simulink model "ctrl"  (R2018a)
settings: Solver=FixedStepDiscrete  StartTime=0.0  StopTime=0.1  RelTol=1e-3  EnableMultiTasking=on
undefined symbols (not defined in the file): AutoCalSt, Cfg_AutoCalEnbl, Cfg_EnblLoadObs, Cfg_IfbkCtrlBW, Cfg_SpdCtrlBW, Cfg_SpdSnsSrc, DiscIntNeverNeededParam, DistObs_K1, DistObs_K2, DistObs_K3, EncResDeg, MotorParams, MtrCtrlMd, SmDiff_Ki, SmDiff_Kp, TsFast
libraries: ctrl_lib x9, simulink_extras x4, simulink x3, adrc_lib x1
settings Model: PauseTimes=0.1  Creator=uids8840  LastModifiedBy=elrobotista
settings SolverCC: AutoInsertRateTranBlk=on
settings DataIOCC: SaveOutput=off  SignalLogging=off  DSMLogging=off  SaveTime=off
settings OptimizationCC: UseFloatMulNetSlope=on  PassReuseOutputArgsAs=Individual arguments  ZeroExternalMemoryAtStartup=off  ZeroInternalMemoryAtStartup=off  NoFixptDivByZeroProtection=on  EfficientFloat2IntCast=on  LifeSpan=1
settings DebuggingCC: ParameterTunabilityLossMsg=error
settings HardwareCC: ProdBitPerPointer=32  ProdBitPerSizeT=32  ProdBitPerPtrDiffT=32  ProdLargestAtomicInteger=Long  ProdLargestAtomicFloat=Double  ProdWordSize=32  ProdHWDeviceType=ARM Compatible->ARM Cortex
settings ModelReferenceCC: ModelReferenceNumInstancesAllowed=Single
settings SFSimCC: MATLABDynamicMemAlloc=off
settings RTWCC: SystemTargetFile=ert.tlc  GenCodeOnly=on  PackageGeneratedCodeAndArtifacts=on  PackageName=mtrctl  TemplateMakefile=ert_default_tmf  GenerateReport=on  IncludeHyperlinkInReport=on  LaunchReport=on  GenerateTraceInfo=on  GenerateTraceReport=on  GenerateTraceReportSl=on  GenerateTraceReportSf=on  GenerateTraceReportEml=on  GenerateCodeMetricsReport=on
settings CodeAppCC: ForceParamTrailComments=on  IgnoreCustomStorageClasses=off  OperatorAnnotations=on  SimulinkDataObjDesc=on  SFDataObjDesc=on  CustomSymbolStrGlobalVar=rt$N$M  CustomSymbolStrType=$N$M  CustomSymbolStrFcn=$N$M$F  CustomSymbolStrMacro=$N$M  InsertBlockDesc=on
settings ERTTargetCC: TargetLangStandard=C99 (ISO)  GenerateFullHeader=off  IncludeMdlTerminateFcn=off  CombineSignalStateStructs=on  SuppressErrorStatus=on  ERTCustomFileBanners=off  SupportAbsoluteTime=off  SupportNonFinite=off  SupportComplex=off  ERTCustomFileTemplate=example_file_process.tlc

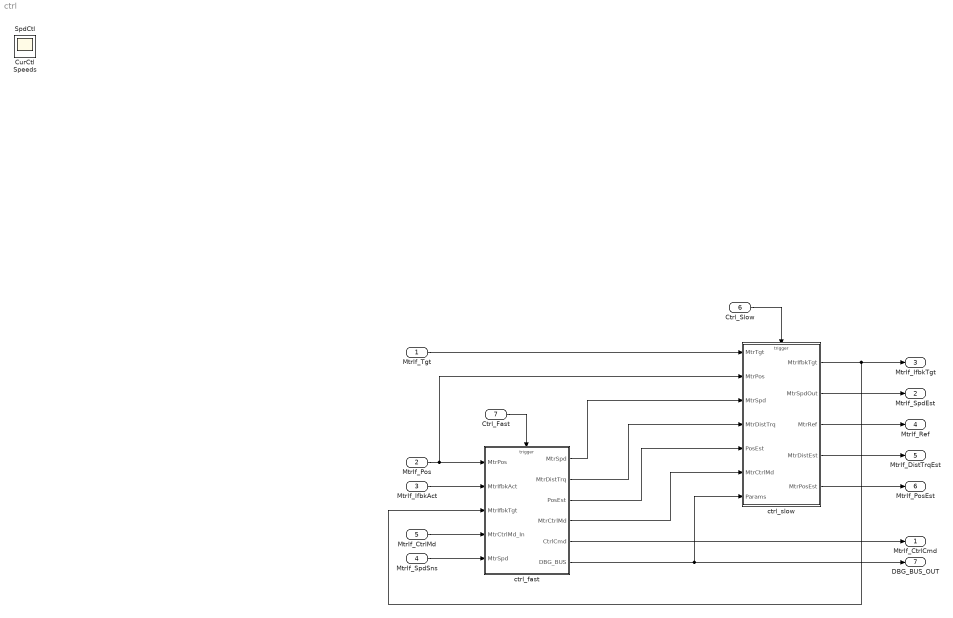
== system ctrl ==
  MtrIf_Tgt : Inport  OutDataTypeStr=single
  MtrIf_Pos : Inport  Port=2  OutDataTypeStr=single
  MtrIf_IfbkAct : Inport  Port=3  OutDataTypeStr=single
  MtrIf_SpdSns : Inport  Port=4
  MtrIf_CtrlMd : Inport  Port=5  OutDataTypeStr=Enum: MtrCtrlMd
  Ctrl_Slow : Inport  Port=6  OutputFunctionCall=on
  Ctrl_Fast : Inport  Port=7  OutputFunctionCall=on
  ctrl_fast : Subsystem  TreatAsAtomicUnit=on  SystemSampleTime=1/30e3
      settings: RTWFcnNameOpts=Use subsystem name  RTWFileNameOpts=Use subsystem name  FunctionInterfaceSpec=Allow arguments
  ctrl_slow : Subsystem  TreatAsAtomicUnit=on  SystemSampleTime=1/1e3
      settings: RTWFcnNameOpts=Use subsystem name  RTWFileNameOpts=Use function name  FunctionInterfaceSpec=Allow arguments
  MtrIf_CtrlCmd : Outport
  MtrIf_SpdEst : Outport  Port=2
  MtrIf_IfbkTgt : Outport  Port=3
  MtrIf_Ref : Outport  Port=4
  MtrIf_DistTrqEst : Outport  Port=5
  MtrIf_PosEst : Outport  Port=6
  DBG_BUS_OUT : Outport  Port=7  OutDataTypeStr=Bus: DBG_BUS  BusOutputAsStruct=on
  CurCtl : Scope
  SpdCtl : Scope
  Speeds : Scope
  wires:
  ctrl_fast/1(MtrSpd) -> ctrl_slow/3(MtrSpd)
  Ctrl_Slow/1 -> ctrl_slow/Trigger
  Ctrl_Fast/1 -> ctrl_fast/Trigger
  MtrIf_IfbkAct/1 -> ctrl_fast/2(MtrIfbkAct)
  MtrIf_Pos/1 -> ctrl_fast/1(" MtrPos"), ctrl_slow/2(MtrPos)
  ctrl_slow/2(MtrSpdOut) -> MtrIf_SpdEst/1
  ctrl_slow/1(MtrIfbkTgt) -> MtrIf_IfbkTgt/1, ctrl_fast/3(MtrIfbkTgt)
  MtrIf_Tgt/1 -> ctrl_slow/1(MtrTgt)
  ctrl_slow/3(MtrRef) -> MtrIf_Ref/1
  ctrl_slow/4(MtrDistEst) -> MtrIf_DistTrqEst/1
  ctrl_slow/5(MtrPosEst) -> MtrIf_PosEst/1
  ctrl_fast/5(CtrlCmd) -> MtrIf_CtrlCmd/1
  ctrl_fast/2(MtrDistTrq) -> ctrl_slow/4(MtrDistTrq)
  ctrl_fast/3(PosEst) -> ctrl_slow/5(PosEst)
  MtrIf_CtrlMd/1 -> ctrl_fast/4(MtrCtrlMd_In)
  MtrIf_SpdSns/1 -> ctrl_fast/5(" MtrSpd")
  ctrl_fast/4(MtrCtrlMd) -> ctrl_slow/6(MtrCtrlMd)
  ctrl_fast/6(DBG_BUS) -> ctrl_slow/7(Params), DBG_BUS_OUT/1

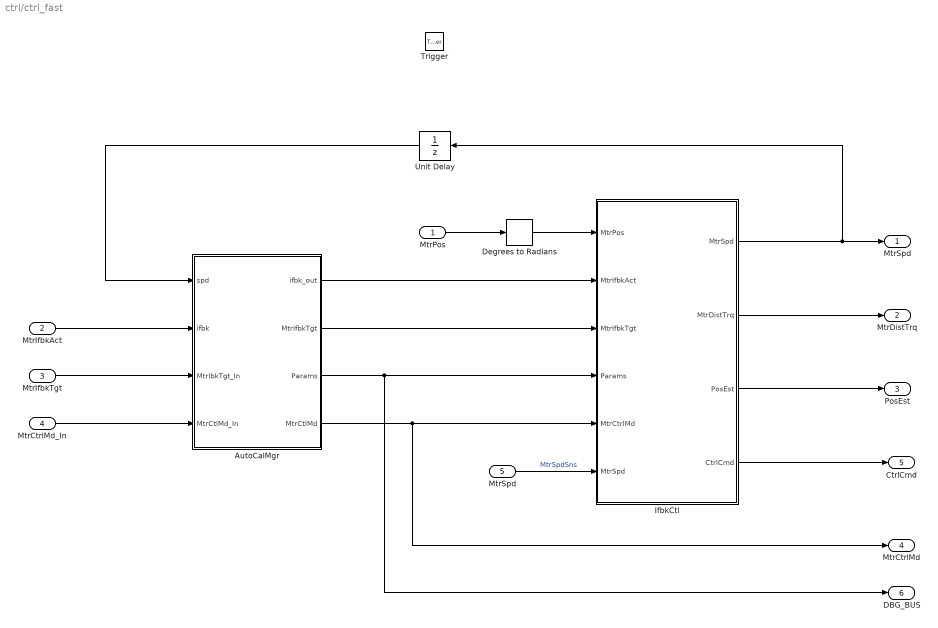
== system ctrl/ctrl_fast ==
  " MtrPos" : Inport
  MtrIfbkAct : Inport  Port=2
  MtrIfbkTgt : Inport  Port=3
  MtrCtrlMd_In : Inport  Port=4
  " MtrSpd" : Inport  Port=5
  Trigger : TriggerPort  TriggerType=function-call  VariantControl=Variant  PortDimensions=1
  AutoCalMgr : Subsystem
  Degrees to Radians : simulink_extras/Transformations/Degrees to Radians
  IfbkCtl : Subsystem
  Unit Delay : UnitDelay  SampleTime=-1
  MtrSpd : Outport
  MtrDistTrq : Outport  Port=2
  PosEst : Outport  Port=3
  MtrCtrlMd : Outport  Port=4
  CtrlCmd : Outport  Port=5
  DBG_BUS : Outport  Port=6  OutDataTypeStr=Bus: DBG_BUS
  wires:
  " MtrSpd"/1 -> IfbkCtl/6(" MtrSpd")  "MtrSpdSns"
  IfbkCtl/2(MtrDistTrq) -> MtrDistTrq/1
  IfbkCtl/4(CtrlCmd) -> CtrlCmd/1
  MtrIfbkAct/1 -> AutoCalMgr/2(ifbk)
  MtrIfbkTgt/1 -> AutoCalMgr/3(MtrIbkTgt_In)
  AutoCalMgr/1(ifbk_out) -> IfbkCtl/2(MtrIfbkAct)
  AutoCalMgr/2(MtrIfbkTgt) -> IfbkCtl/3(MtrIfbkTgt)
  AutoCalMgr/4(MtrCtlMd) -> MtrCtrlMd/1, IfbkCtl/5(MtrCtrlMd)
  MtrCtrlMd_In/1 -> AutoCalMgr/4(MtrCtlMd_In)
  AutoCalMgr/3(Params) -> DBG_BUS/1, IfbkCtl/4(Params)
  IfbkCtl/1(MtrSpd) -> Unit Delay/1, MtrSpd/1
  Unit Delay/1 -> AutoCalMgr/1(spd)
  " MtrPos"/1 -> Degrees to Radians/1
  Degrees to Radians/1 -> IfbkCtl/1(" MtrPos")
  IfbkCtl/3(PosEst) -> PosEst/1

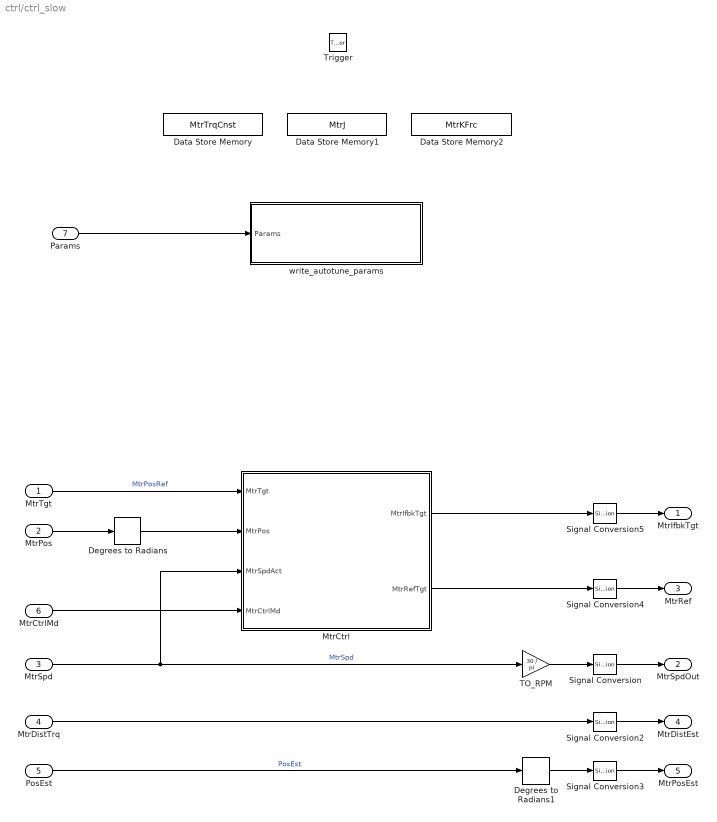
== system ctrl/ctrl_slow ==
  MtrTgt : Inport
  MtrPos : Inport  Port=2
  MtrSpd : Inport  Port=3
  MtrDistTrq : Inport  Port=4
  PosEst : Inport  Port=5
  MtrCtrlMd : Inport  Port=6
  Params : Inport  Port=7  OutDataTypeStr=Bus: DBG_BUS
  Trigger : TriggerPort  TriggerType=function-call  VariantControl=Variant  PortDimensions=1
  Data Store Memory : DataStoreMemory  DataStoreName=MtrTrqCnst  ReadBeforeWriteMsg=warning  WriteAfterWriteMsg=warning  WriteAfterReadMsg=warning  ShowAdditionalParam=off
  Data Store Memory1 : DataStoreMemory  DataStoreName=MtrJ  ReadBeforeWriteMsg=warning  WriteAfterWriteMsg=warning  WriteAfterReadMsg=warning  ShowAdditionalParam=off
  Data Store Memory2 : DataStoreMemory  DataStoreName=MtrKFrc  ReadBeforeWriteMsg=warning  WriteAfterWriteMsg=warning  WriteAfterReadMsg=warning  ShowAdditionalParam=off
  Degrees to Radians : simulink_extras/Transformations/Degrees to Radians
  Degrees to Radians1 : simulink_extras/Transformations/Degrees to Radians
  MtrCtrl : Subsystem
  Signal Conversion{,2..5} (5 alike) : SignalConversion  OverrideOpt=off
  TO_RPM : Gain  Gain=30 / pi
  write_autotune_params : Subsystem
  MtrIfbkTgt : Outport
  MtrSpdOut : Outport  Port=2
  MtrRef : Outport  Port=3
  MtrDistEst : Outport  Port=4
  MtrPosEst : Outport  Port=5
  wires:
  MtrCtrl/1(MtrIfbkTgt) -> Signal Conversion5/1
  Signal Conversion5/1 -> MtrIfbkTgt/1
  Signal Conversion/1 -> MtrSpdOut/1
  PosEst/1 -> Degrees to Radians1/1  "PosEst"
  Signal Conversion2/1 -> MtrDistEst/1
  Signal Conversion3/1 -> MtrPosEst/1
  Signal Conversion4/1 -> MtrRef/1
  MtrTgt/1 -> MtrCtrl/1(MtrTgt)  "MtrPosRef"
  MtrCtrlMd/1 -> MtrCtrl/4(MtrCtrlMd)
  MtrDistTrq/1 -> Signal Conversion2/1
  MtrPos/1 -> Degrees to Radians/1
  MtrCtrl/2(MtrRefTgt) -> Signal Conversion4/1
  Params/1 -> write_autotune_params/1(Params)
  Degrees to Radians/1 -> MtrCtrl/2(MtrPos)
  Degrees to Radians1/1 -> Signal Conversion3/1
  TO_RPM/1 -> Signal Conversion/1
  MtrSpd/1 -> MtrCtrl/3(MtrSpdAct), TO_RPM/1  "MtrSpd"

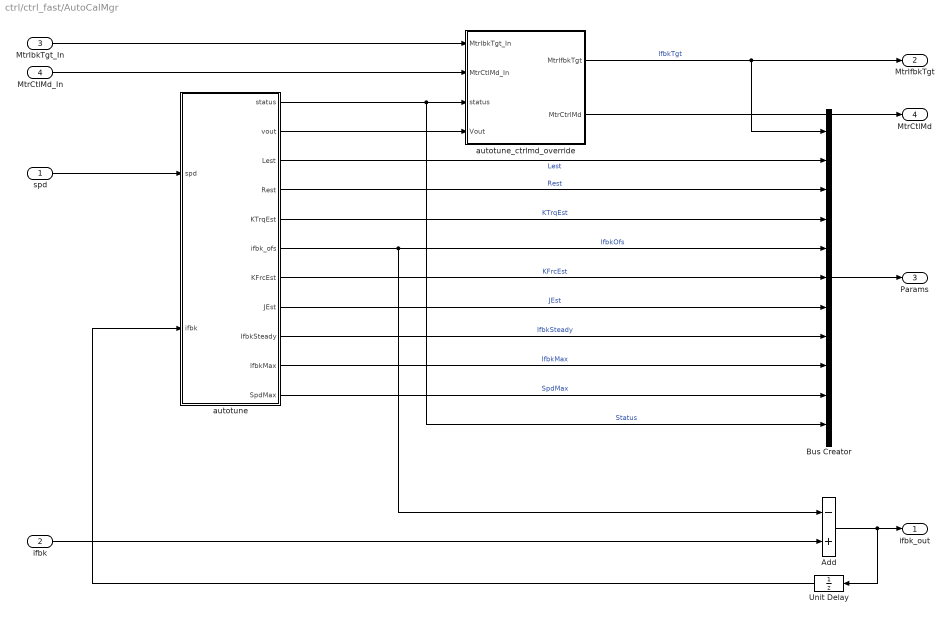
== system ctrl/ctrl_fast/AutoCalMgr ==
  spd : Inport
  ifbk : Inport  Port=2
  MtrIbkTgt_In : Inport  Port=3
  MtrCtlMd_In : Inport  Port=4
  Add : Sum  Inputs=-+
  Bus Creator : BusCreator  Inputs=11  OutDataTypeStr=Bus: DBG_BUS  NonVirtualBus=on
  Unit Delay : UnitDelay  SampleTime=-1
  autotune : Stateflow chart  TreatAsAtomicUnit=on
  autotune_ctrlmd_override : Subsystem
  ifbk_out : Outport
  MtrIfbkTgt : Outport  Port=2
  Params : Outport  Port=3
  MtrCtlMd : Outport  Port=4
  wires:
  MtrIbkTgt_In/1 -> autotune_ctrlmd_override/1(MtrIbkTgt_In)
  MtrCtlMd_In/1 -> autotune_ctrlmd_override/2(MtrCtlMd_In)
  autotune_ctrlmd_override/1(MtrIfbkTgt) -> Bus Creator/1, MtrIfbkTgt/1  "IfbkTgt"
  autotune_ctrlmd_override/2(MtrCtrlMd) -> MtrCtlMd/1
  autotune/1(status) -> Bus Creator/11, autotune_ctrlmd_override/3(status)  "Status"
  autotune/2(vout) -> autotune_ctrlmd_override/4(Vout)
  Bus Creator/1 -> Params/1
  ifbk/1 -> Add/2
  spd/1 -> autotune/1(spd)
  autotune/6(ifbk_ofs) -> Bus Creator/5, Add/1  "IfbkOfs"
  Add/1 -> Unit Delay/1, ifbk_out/1
  Unit Delay/1 -> autotune/2(ifbk)
  autotune/3(Lest) -> Bus Creator/2  "Lest"
  autotune/4(Rest) -> Bus Creator/3  "Rest"
  autotune/5(KTrqEst) -> Bus Creator/4  "KTrqEst"
  autotune/7(KFrcEst) -> Bus Creator/6  "KFrcEst"
  autotune/8(JEst) -> Bus Creator/7  "JEst"
  autotune/9(IfbkSteady) -> Bus Creator/8  "IfbkSteady"
  autotune/10(IfbkMax) -> Bus Creator/9  "IfbkMax"
  autotune/11(SpdMax) -> Bus Creator/10  "SpdMax"

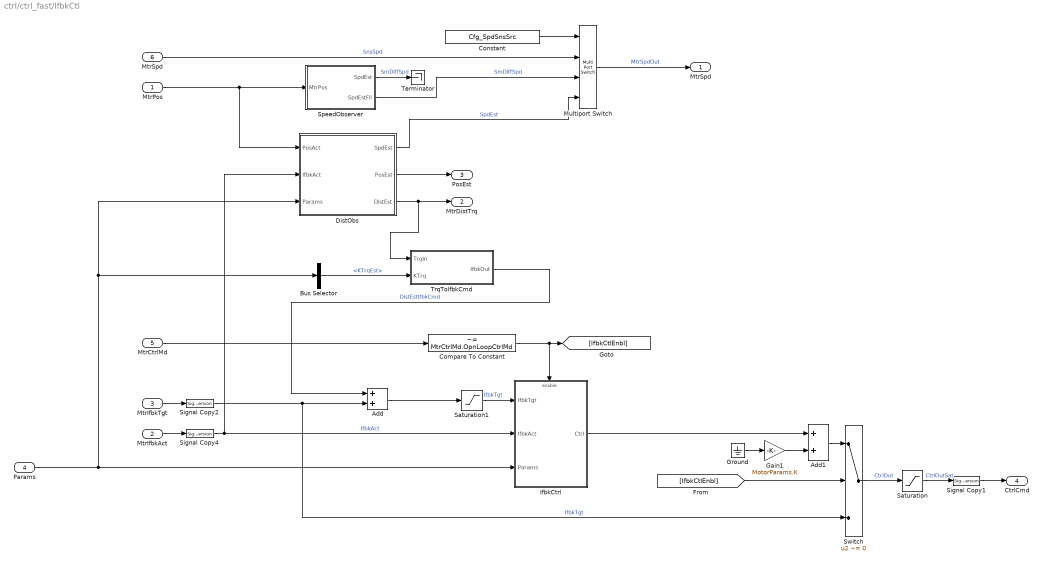
== system ctrl/ctrl_fast/IfbkCtl ==
  " MtrPos" : Inport
  MtrIfbkAct : Inport  Port=2
  MtrIfbkTgt : Inport  Port=3
  Params : Inport  Port=4
  MtrCtrlMd : Inport  Port=5
  " MtrSpd" : Inport  Port=6
  Add : Sum
  Add1 : Sum
  Bus Selector : BusSelector  OutputSignals=KTrqEst
  Compare To Constant : simulink/Logic and Bit Operations/Compare To Constant  relop=~=  const=MtrCtrlMd.OpnLoopCtrlMd  OutDataTypeStr=boolean
  Constant : Constant  Value=Cfg_SpdSnsSrc
  DistObs : Subsystem
  Gain1 : Gain  Gain=MotorParams.K
      settings: AttributesFormatString=%<Gain>
  Ground : Ground
  IfbkCtrl : Subsystem
  Multiport Switch : MultiPortSwitch  DataPortOrder=Zero-based contiguous  DiagnosticForDefault=None  zeroidx=on
  Saturation : Saturate  UpperLimit=12  LowerLimit=-12
  Saturation1 : Saturate  UpperLimit=0.6  LowerLimit=-0.6
  Signal Copy1 : SignalConversion  OverrideOpt=off
  Signal Copy2 : SignalConversion  OverrideOpt=off
  Signal Copy4 : SignalConversion  OverrideOpt=off
  SpeedObserver : Subsystem  RTWFcnName=SpdEst  RTWFileName=spdest
      settings: RTWFcnNameOpts=Use subsystem name  RTWFileNameOpts=Use subsystem name
  Switch : Switch  Criteria=u2 ~= 0
  Terminator : Terminator
  TrqToIfbkCmd : Subsystem
  MtrSpd : Outport
  MtrDistTrq : Outport  Port=2
  PosEst : Outport  Port=3
  CtrlCmd : Outport  Port=4
  wires:
  IfbkCtrl/1(Ctrl) -> Add1/1
  Compare To Constant/1 -> [IfbkCtlEnbl], IfbkCtrl/Enable
  MtrIfbkTgt/1 -> Signal Copy2/1
  MtrCtrlMd/1 -> Compare To Constant/1
  Add1/1 -> Switch/1
  Signal Copy4/1 -> DistObs/2(IfbkAct), IfbkCtrl/2(IfbkAct)  "IfbkAct"
  Gain1/1 -> Add1/2
  Multiport Switch/1 -> MtrSpd/1  "MtrSpdOut"
  Switch/1 -> Saturation/1  "CtrlOut"
  MtrIfbkAct/1 -> Signal Copy4/1
  " MtrSpd"/1 -> Multiport Switch/2  "SnsSpd"
  Constant/1 -> Multiport Switch/1
  [IfbkCtlEnbl] -> Switch/2
  Signal Copy2/1 -> Add/2, Switch/3  "IfbkTgt"
  SpeedObserver/2(SpdEstFil) -> Multiport Switch/3  "SmDiffSpd"
  " MtrPos"/1 -> DistObs/1(PosAct), SpeedObserver/1(MtrPos)
  Ground/1 -> Gain1/1
  Saturation/1 -> Signal Copy1/1  "CtrlOutSat"
  Signal Copy1/1 -> CtrlCmd/1
  Params/1 -> DistObs/3(Params), Bus Selector/1, IfbkCtrl/3(Params)
  SpeedObserver/1(SpdEst) -> Terminator/1  "SmDiffSpd"
  Saturation1/1 -> IfbkCtrl/1(IfbkTgt)  "IfbkTgt"
  TrqToIfbkCmd/1(IfbkOut) -> Add/1  "DistEstIfbkCmd"
  Add/1 -> Saturation1/1
  DistObs/3(DistEst) -> MtrDistTrq/1, TrqToIfbkCmd/1(TrqIn)
  DistObs/1(SpdEst) -> Multiport Switch/4  "SpdEst"
  DistObs/2(PosEst) -> PosEst/1
  Bus Selector/1 -> TrqToIfbkCmd/2(KTrq)  "<KTrqEst>"

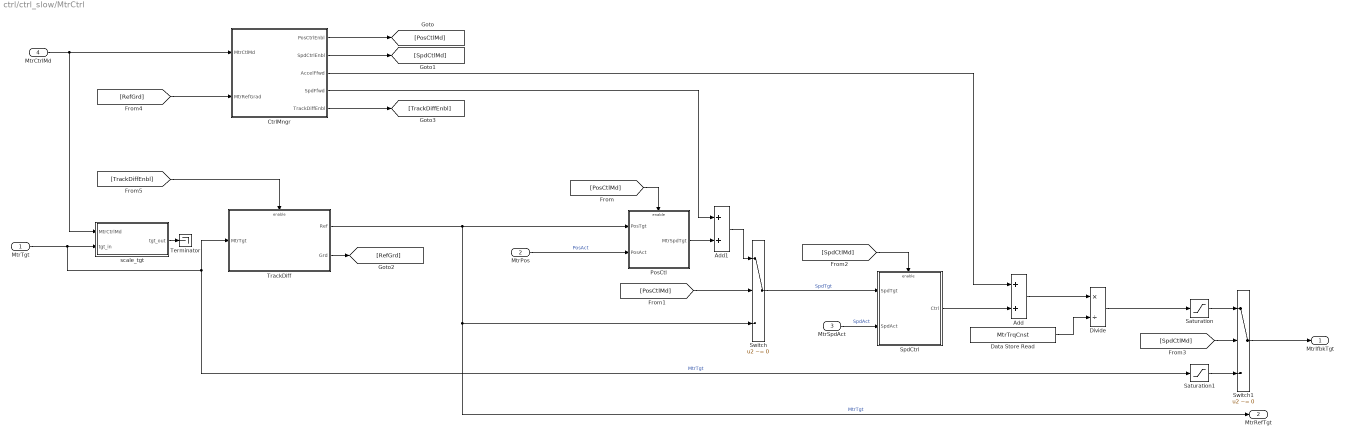
== system ctrl/ctrl_slow/MtrCtrl ==
  MtrTgt : Inport
  MtrPos : Inport  Port=2
  MtrSpdAct : Inport  Port=3
  MtrCtrlMd : Inport  Port=4
  Add : Sum
  Add1 : Sum
  CtrlMngr : Subsystem
  Data Store Read : DataStoreRead  DataStoreName=MtrTrqCnst
  Divide : Product  Inputs=*/
  PosCtl : Subsystem
  Saturation : Saturate
  Saturation1 : Saturate  UpperLimit=12  LowerLimit=-12
  SpdCtrl : Subsystem
  Switch : Switch  Criteria=u2 ~= 0
  Switch1 : Switch  Criteria=u2 ~= 0
  Terminator : Terminator
  TrackDiff : Subsystem  AncestorBlock=adrc_lib/TrackDiff  mask{ts=1e-3, h0=1e-3, r0=200}
      mask prompts: ts "Exeuction rate [s]:"
  scale_tgt : Subsystem
  MtrIfbkTgt : Outport
  MtrRefTgt : Outport  Port=2
  wires:
  MtrPos/1 -> PosCtl/2(PosAct)  "PosAct"
  TrackDiff/1(Ref) -> PosCtl/1(PosTgt), Switch/3, MtrRefTgt/1  "MtrTgt"
  [PosCtlMd] -> PosCtl/Enable
  [PosCtlMd] -> Switch/2
  Switch/1 -> SpdCtrl/1(SpdTgt)  "SpdTgt"
  MtrSpdAct/1 -> SpdCtrl/2(SpdAct)  "SpdAct"
  [SpdCtlMd] -> SpdCtrl/Enable
  [SpdCtlMd] -> Switch1/2
  Add/1 -> Divide/1
  SpdCtrl/1(Ctrl) -> Add/2
  PosCtl/1(MtrSpdTgt) -> Add1/2
  Add1/1 -> Switch/1
  MtrCtrlMd/1 -> scale_tgt/1(MtrCtrlMd), CtrlMngr/1(MtrCtlMd)
  [RefGrd] -> CtrlMngr/2(MtrRefGrad)
  CtrlMngr/1(PosCtrlEnbl) -> [PosCtlMd]
  CtrlMngr/2(SpdCtrlEnbl) -> [SpdCtlMd]
  CtrlMngr/3(AccelFfwd) -> Add/1
  CtrlMngr/4(SpdFfwd) -> Add1/1
  TrackDiff/2(Grd) -> [RefGrd]
  CtrlMngr/5(TrackDiffEnbl) -> [TrackDiffEnbl]
  [TrackDiffEnbl] -> TrackDiff/Enable
  Switch1/1 -> MtrIfbkTgt/1
  Divide/1 -> Saturation/1
  MtrTgt/1 -> TrackDiff/1(MtrTgt), Saturation1/1, scale_tgt/2(tgt_in)  "MtrTgt"
  Saturation/1 -> Switch1/1
  Saturation1/1 -> Switch1/3
  Data Store Read/1 -> Divide/2
  scale_tgt/1(tgt_out) -> Terminator/1

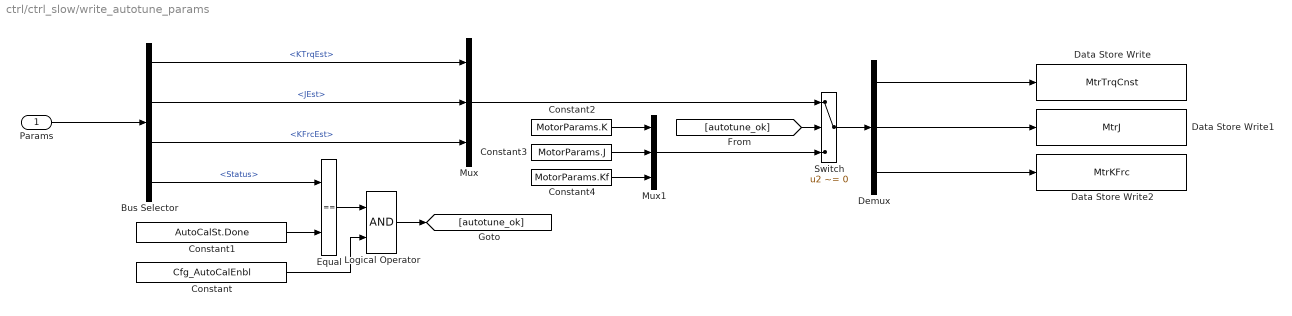
== system ctrl/ctrl_slow/write_autotune_params ==
  Params : Inport
  Bus Selector : BusSelector  OutputSignals=KTrqEst,JEst,KFrcEst,Status
  Constant : Constant  Value=Cfg_AutoCalEnbl
  Constant1 : Constant  Value=AutoCalSt.Done  OutDataTypeStr=Enum: AutoCalSt
  Constant2 : Constant  Value=MotorParams.K  OutDataTypeStr=Inherit: Inherit via back propagation
  Constant3 : Constant  Value=MotorParams.J  OutDataTypeStr=Inherit: Inherit via back propagation
  Constant4 : Constant  Value=MotorParams.Kf  OutDataTypeStr=Inherit: Inherit via back propagation
  Data Store Write : DataStoreWrite  DataStoreName=MtrTrqCnst
  Data Store Write1 : DataStoreWrite  DataStoreName=MtrJ
  Data Store Write2 : DataStoreWrite  DataStoreName=MtrKFrc
  Demux : Demux  Outputs=3
  Equal : RelationalOperator  Operator===  OutDataTypeStr=boolean  RndMeth=Simplest
  Logical Operator : Logic  AllPortsSameDT=off  OutDataTypeStr=boolean
  Mux : Mux  Inputs=3
  Mux1 : Mux  Inputs=3
  Switch : Switch  Criteria=u2 ~= 0
  wires:
  Bus Selector/1 -> Mux/1  "<KTrqEst>"
  Bus Selector/3 -> Mux/3  "<KFrcEst>"
  Params/1 -> Bus Selector/1
  Bus Selector/2 -> Mux/2  "<JEst>"
  Bus Selector/4 -> Equal/1  "<Status>"
  Constant1/1 -> Equal/2
  Equal/1 -> Logical Operator/1
  Constant/1 -> Logical Operator/2
  Logical Operator/1 -> [autotune_ok]
  [autotune_ok] -> Switch/2
  Mux/1 -> Switch/1
  Mux1/1 -> Switch/3
  Constant2/1 -> Mux1/1
  Constant3/1 -> Mux1/2
  Constant4/1 -> Mux1/3
  Switch/1 -> Demux/1
  Demux/2 -> Data Store Write1/1
  Demux/1 -> Data Store Write/1
  Demux/3 -> Data Store Write2/1

== system ctrl/ctrl_fast/AutoCalMgr/autotune_ctrlmd_override ==
  MtrIbkTgt_In : Inport
  MtrCtlMd_In : Inport  Port=2
  status : Inport  Port=3
  Vout : Inport  Port=4
  Constant : Constant  Value=MtrCtrlMd.OpnLoopCtrlMd  OutDataTypeStr=Inherit: Inherit via back propagation
  Switch : Switch  Criteria=u2 ~= 0
  Switch1 : Switch  Criteria=u2 ~= 0
  autocal_override : Subsystem
  MtrIfbkTgt : Outport
  MtrCtrlMd : Outport  Port=2
  wires:
  Constant/1 -> Switch1/3
  MtrIbkTgt_In/1 -> Switch/1
  status/1 -> autocal_override/1(AutoCalSt)
  Vout/1 -> Switch/3
  autocal_override/1(OverrideNotActv) -> Switch/2, Switch1/2
  MtrCtlMd_In/1 -> Switch1/1
  Switch/1 -> MtrIfbkTgt/1
  Switch1/1 -> MtrCtrlMd/1

== system ctrl/ctrl_fast/IfbkCtl/DistObs ==
  PosAct : Inport
  IfbkAct : Inport  Port=2
  Params : Inport  Port=3
  Bus Selector : BusSelector  OutputSignals=KTrqEst,JEst,KFrcEst
  DistObsJ : Subsystem  AncestorBlock=adrc_lib/DistObsJ  SystemSampleTime=1/30e3  mask{ts=TsFast, k1=DistObs_K1, k2=DistObs_K2, k3=DistObs_K3}
      mask prompts: ts "Execution rate [s]"; k1 "Gain K1:"; k2 "Gain K2:"; k3 "Gain K3:"
  Product : Product
  SpdEst : Outport
  PosEst : Outport  Port=2
  DistEst : Outport  Port=3
  wires:
  PosAct/1 -> DistObsJ/1(MtrPosAct)
  DistObsJ/3(MtrDistEst) -> DistEst/1  "DistEst"
  DistObsJ/1(MtrPosEst) -> PosEst/1
  IfbkAct/1 -> Product/1
  DistObsJ/2(MtrSpdEst) -> SpdEst/1  "DistObsSpd"
  Params/1 -> Bus Selector/1
  Bus Selector/1 -> Product/2  "<KTrqEst>"
  Product/1 -> DistObsJ/2(MtrTrqAct)
  Bus Selector/2 -> DistObsJ/3(MtrJ)  "<JEst>"
  Bus Selector/3 -> DistObsJ/4(MtrKFrc)  "<KFrcEst>"

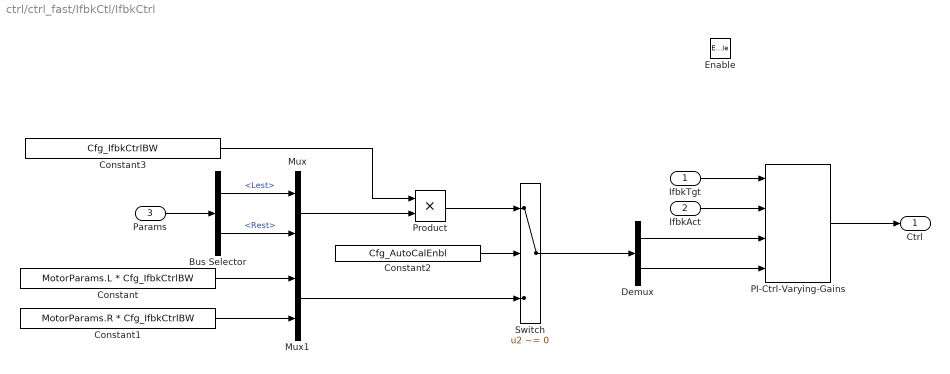
== system ctrl/ctrl_fast/IfbkCtl/IfbkCtrl ==
  IfbkTgt : Inport
  IfbkAct : Inport  Port=2
  Params : Inport  Port=3
  Enable : EnablePort  StatesWhenEnabling=reset
  Bus Selector : BusSelector  OutputSignals=Lest,Rest
  Constant : Constant  Value=MotorParams.L * Cfg_IfbkCtrlBW
  Constant1 : Constant  Value=MotorParams.R * Cfg_IfbkCtrlBW
  Constant2 : Constant  Value=Cfg_AutoCalEnbl
  Constant3 : Constant  Value=Cfg_IfbkCtrlBW
  Demux : Demux  Outputs=2
  Mux : Mux  Inputs=2
  Mux1 : Mux  Inputs=2
  PI-Ctrl-Varying-Gains : ctrl_lib/PI-Ctrl-Varying-Gains  ts=TsFast  max_lim=12  min_lim=-12
  Product : Product
  Switch : Switch  Criteria=u2 ~= 0
  Ctrl : Outport
  wires:
  IfbkTgt/1 -> PI-Ctrl-Varying-Gains/1
  IfbkAct/1 -> PI-Ctrl-Varying-Gains/2
  PI-Ctrl-Varying-Gains/1 -> Ctrl/1
  Params/1 -> Bus Selector/1
  Bus Selector/2 -> Mux/2  "<Rest>"
  Bus Selector/1 -> Mux/1  "<Lest>"
  Demux/1 -> PI-Ctrl-Varying-Gains/3
  Demux/2 -> PI-Ctrl-Varying-Gains/4
  Constant/1 -> Mux1/1
  Constant1/1 -> Mux1/2
  Switch/1 -> Demux/1
  Mux/1 -> Product/2
  Constant2/1 -> Switch/2
  Mux1/1 -> Switch/3
  Product/1 -> Switch/1
  Constant3/1 -> Product/1

== system ctrl/ctrl_fast/IfbkCtl/SpeedObserver ==
  MtrPos : Inport
  D-1LPF : ctrl_lib/D-1LPF  k_filt=SmDiff_FiltCnst
  SM-Differentiator : Subsystem  AncestorBlock=ctrl_lib/SM-Differentiator  mask{sm_ki=SmDiff_Ki, sm_kp=SmDiff_Kp, ts=TsFast}
      mask prompts: sm_ki "Integral Gain:"; sm_kp "Proportional Gain:"; ts "Execution Rate [s]:"
      mask DialogControl DescTextVar Prompt: Second order sliding mode differentiator.
  Signal Conversion : SignalConversion  OverrideOpt=off
  SpdEst : Outport
  SpdEstFil : Outport  Port=2
  wires:
  SM-Differentiator/1(DiffOut) -> SpdEst/1, D-1LPF/1
  D-1LPF/1 -> Signal Conversion/1
  MtrPos/1 -> SM-Differentiator/1(DiffIn)
  Signal Conversion/1 -> SpdEstFil/1

== system ctrl/ctrl_fast/IfbkCtl/TrqToIfbkCmd ==
  TrqIn : Inport
  KTrq : Inport  Port=2
  Constant1 : Constant  Value=Cfg_EnblLoadObs
  Constant2 : Constant  Value=0  OutDataTypeStr=Inherit: Inherit via back propagation
  Divide : Product  Inputs=*/
  Switch2 : Switch  Criteria=u2 ~= 0
  IfbkOut : Outport
  wires:
  Constant2/1 -> Switch2/3
  KTrq/1 -> Divide/2
  Constant1/1 -> Switch2/2
  Divide/1 -> Switch2/1
  TrqIn/1 -> Divide/1
  Switch2/1 -> IfbkOut/1

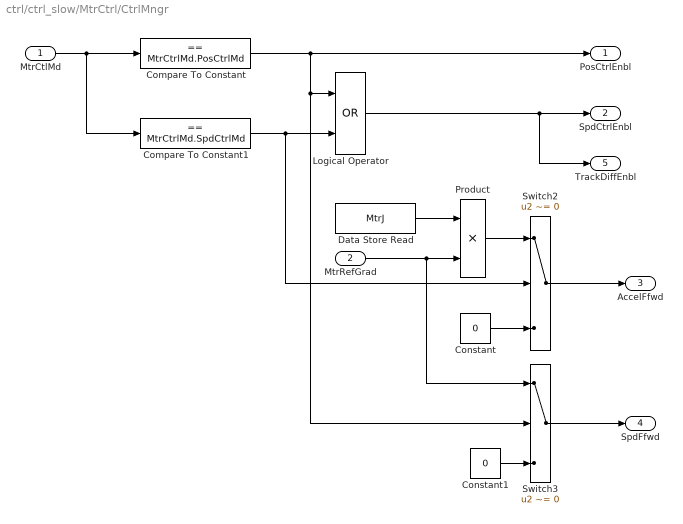
== system ctrl/ctrl_slow/MtrCtrl/CtrlMngr ==
  MtrCtlMd : Inport
  MtrRefGrad : Inport  Port=2
  Compare To Constant : simulink/Logic and Bit Operations/Compare To Constant  relop===  const=MtrCtrlMd.PosCtrlMd  OutDataTypeStr=boolean
  Compare To Constant1 : simulink/Logic and Bit Operations/Compare To Constant  relop===  const=MtrCtrlMd.SpdCtrlMd  OutDataTypeStr=boolean
  Constant : Constant  Value=0  OutDataTypeStr=Inherit: Inherit via back propagation
  Constant1 : Constant  Value=0  OutDataTypeStr=Inherit: Inherit via back propagation
  Data Store Read : DataStoreRead  DataStoreName=MtrJ
  Logical Operator : Logic  Operator=OR  AllPortsSameDT=off  OutDataTypeStr=boolean
  Product : Product
  Switch2 : Switch  Criteria=u2 ~= 0
  Switch3 : Switch  Criteria=u2 ~= 0
  PosCtrlEnbl : Outport
  SpdCtrlEnbl : Outport  Port=2
  AccelFfwd : Outport  Port=3
  SpdFfwd : Outport  Port=4
  TrackDiffEnbl : Outport  Port=5
  wires:
  Product/1 -> Switch2/1
  Compare To Constant1/1 -> Logical Operator/2, Switch2/2
  Constant1/1 -> Switch3/3
  MtrRefGrad/1 -> Switch3/1, Product/2
  Compare To Constant/1 -> PosCtrlEnbl/1, Switch3/2, Logical Operator/1
  Switch3/1 -> SpdFfwd/1
  Switch2/1 -> AccelFfwd/1
  Constant/1 -> Switch2/3
  MtrCtlMd/1 -> Compare To Constant1/1, Compare To Constant/1
  Logical Operator/1 -> TrackDiffEnbl/1, SpdCtrlEnbl/1
  Data Store Read/1 -> Product/1

== system ctrl/ctrl_slow/MtrCtrl/PosCtl ==
  PosTgt : Inport
  PosAct : Inport  Port=2
  Enable : EnablePort  StatesWhenEnabling=reset
  PI-Ctrl : ctrl_lib/PI-Ctrl  ts=TsMain  PI_Kp=PosCtrl_Kp  PI_Ki=0  max_lim=150  min_lim=-150
  MtrSpdTgt : Outport
  wires:
  PI-Ctrl/1 -> MtrSpdTgt/1  "MtrSpdTgt"
  PosTgt/1 -> PI-Ctrl/1
  PosAct/1 -> PI-Ctrl/2

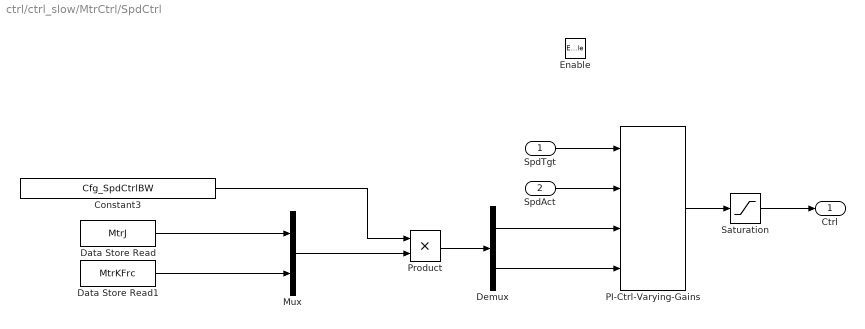
== system ctrl/ctrl_slow/MtrCtrl/SpdCtrl ==
  SpdTgt : Inport
  SpdAct : Inport  Port=2
  Enable : EnablePort  StatesWhenEnabling=reset
  Constant3 : Constant  Value=Cfg_SpdCtrlBW
  Data Store Read : DataStoreRead  DataStoreName=MtrJ
  Data Store Read1 : DataStoreRead  DataStoreName=MtrKFrc
  Demux : Demux  Outputs=2
  Mux : Mux  Inputs=2
  PI-Ctrl-Varying-Gains : ctrl_lib/PI-Ctrl-Varying-Gains  ts=TsFast  max_lim=0.5  min_lim=-0.5
  Product : Product
  Saturation : Saturate
  Ctrl : Outport
  wires:
  SpdTgt/1 -> PI-Ctrl-Varying-Gains/1
  SpdAct/1 -> PI-Ctrl-Varying-Gains/2
  PI-Ctrl-Varying-Gains/1 -> Saturation/1
  Data Store Read1/1 -> Mux/2
  Data Store Read/1 -> Mux/1
  Demux/1 -> PI-Ctrl-Varying-Gains/3
  Demux/2 -> PI-Ctrl-Varying-Gains/4
  Product/1 -> Demux/1
  Mux/1 -> Product/2
  Constant3/1 -> Product/1
  Saturation/1 -> Ctrl/1

== system ctrl/ctrl_slow/MtrCtrl/TrackDiff ==
  MtrTgt : Inport
  Enable : EnablePort  StatesWhenEnabling=reset
  Add : Sum  Inputs=-+
  Discrete-Time Integrator : DiscreteIntegrator  IntegratorMethod=Accumulation: Forward Euler  gainval=ts  SampleTime=-1  ICPrevOutput=DiscIntNeverNeededParam  ICPrevScaledInput=DiscIntNeverNeededParam
  Discrete-Time Integrator1 : DiscreteIntegrator  IntegratorMethod=Accumulation: Forward Euler  gainval=ts  SampleTime=-1  ICPrevOutput=DiscIntNeverNeededParam  ICPrevScaledInput=DiscIntNeverNeededParam
  fhan : adrc_lib/fhan  r0=r0  h0=h0
  Ref : Outport
  Grd : Outport  Port=2
  wires:
  MtrTgt/1 -> Add/1
  Add/1 -> fhan/1
  fhan/1 -> Discrete-Time Integrator/1
  Discrete-Time Integrator/1 -> Grd/1, fhan/2, Discrete-Time Integrator1/1
  Discrete-Time Integrator1/1 -> Add/2, Ref/1

== system ctrl/ctrl_slow/MtrCtrl/scale_tgt ==
  MtrCtrlMd : Inport
  tgt_in : Inport  Port=2
  Degrees to Radians : simulink_extras/Transformations/Degrees to Radians
  Multiport Switch : MultiPortSwitch  DataPortOrder=Specify indices  DataPortIndices={MtrCtrlMd.PosCtrlMd, MtrCtrlMd.SpdCtrlMd}  DataPortForDefault=Additional data port  DiagnosticForDefault=None
  TO_RADpS : Gain  Gain=30 / pi
  encoder_quant : Subsystem
  tgt_out : Outport
  wires:
  MtrCtrlMd/1 -> Multiport Switch/1
  tgt_in/1 -> TO_RADpS/1, Multiport Switch/4, encoder_quant/1(tgt_in)
  Multiport Switch/1 -> tgt_out/1
  encoder_quant/1(tgt_out) -> Degrees to Radians/1
  Degrees to Radians/1 -> Multiport Switch/2
  TO_RADpS/1 -> Multiport Switch/3

== system ctrl/ctrl_fast/AutoCalMgr/autotune_ctrlmd_override/autocal_override ==
  AutoCalSt : Inport
  Constant : Constant  Value=AutoCalSt.Done  OutDataTypeStr=Inherit: Inherit via back propagation
  Constant1 : Constant  Value=AutoCalSt.NotStarted  OutDataTypeStr=Inherit: Inherit via back propagation
  Logical Operator : Logic  Operator=OR  AllPortsSameDT=off  OutDataTypeStr=boolean
  Relational Operator : RelationalOperator  Operator===  OutDataTypeStr=boolean  RndMeth=Simplest
  Relational Operator1 : RelationalOperator  Operator===  OutDataTypeStr=boolean  RndMeth=Simplest
  OverrideNotActv : Outport
  wires:
  Constant1/1 -> Relational Operator/1
  Constant/1 -> Relational Operator1/1
  Relational Operator/1 -> Logical Operator/2
  Relational Operator1/1 -> Logical Operator/1
  Logical Operator/1 -> OverrideNotActv/1
  AutoCalSt/1 -> Relational Operator/2, Relational Operator1/2

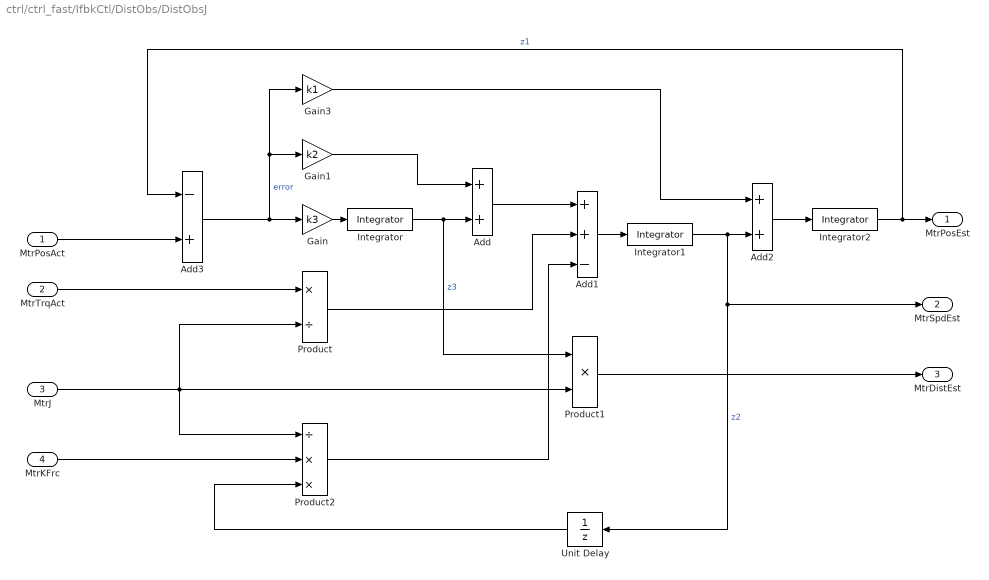
== system ctrl/ctrl_fast/IfbkCtl/DistObs/DistObsJ ==
  MtrPosAct : Inport
  MtrTrqAct : Inport  Port=2
  MtrJ : Inport  Port=3
  MtrKFrc : Inport  Port=4
  Add : Sum
  Add1 : Sum  Inputs=++-
  Add2 : Sum
  Add3 : Sum  Inputs=-+
  Gain : Gain  Gain=k3
      settings: AttributesFormatString=%<Gain>
  Gain1 : Gain  Gain=k2
      settings: AttributesFormatString=%<Gain>
  Gain3 : Gain  Gain=k1
      settings: AttributesFormatString=%<Gain>
  Integrator : ctrl_lib/Integrator  ts=ts  max_lim=1e7  min_lim=-1e7
  Integrator1 : ctrl_lib/Integrator  ts=ts  max_lim=1e7  min_lim=-1e7
  Integrator2 : ctrl_lib/Integrator  ts=ts  max_lim=1e7  min_lim=-1e7
  Product : Product  Inputs=*/
  Product1 : Product  Inputs=**
  Product2 : Product  Inputs=/**
  Unit Delay : UnitDelay  SampleTime=-1
  MtrPosEst : Outport
  MtrSpdEst : Outport  Port=2
  MtrDistEst : Outport  Port=3
  wires:
  MtrJ/1 -> Product2/1, Product1/2, Product/2
  Gain3/1 -> Add2/1
  Add/1 -> Add1/1
  Integrator/1 -> Add/2, Product1/1  "z3"
  Gain1/1 -> Add/1
  Integrator1/1 -> MtrSpdEst/1, Unit Delay/1, Add2/2  "z2"
  Gain/1 -> Integrator/1
  Integrator2/1 -> MtrPosEst/1, Add3/1  "z1"
  Add2/1 -> Integrator2/1
  MtrPosAct/1 -> Add3/2
  Add1/1 -> Integrator1/1
  Product/1 -> Add1/2
  Add3/1 -> Gain3/1, Gain1/1, Gain/1  "error"
  MtrTrqAct/1 -> Product/1
  Product1/1 -> MtrDistEst/1
  Unit Delay/1 -> Product2/3
  MtrKFrc/1 -> Product2/2
  Product2/1 -> Add1/3

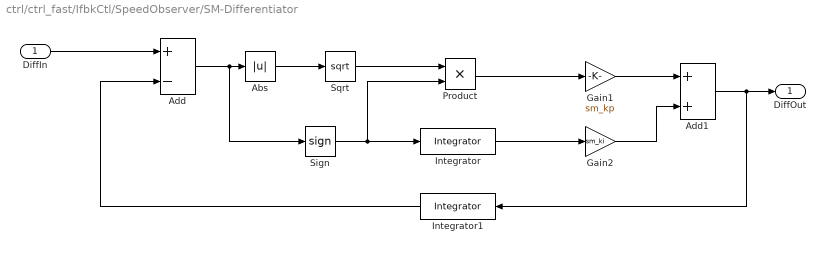
== system ctrl/ctrl_fast/IfbkCtl/SpeedObserver/SM-Differentiator ==
  DiffIn : Inport
  Abs : Abs
  Add : Sum  Inputs=+-
  Add1 : Sum  OutDataTypeStr=Inherit: Inherit via back propagation
  Gain1 : Gain  Gain=sm_kp  ParamDataTypeStr=Inherit: Inherit from 'Gain'  OutDataTypeStr=Inherit: Inherit via back propagation
  Gain2 : Gain  Gain=sm_ki  ParamDataTypeStr=Inherit: Inherit from 'Gain'  OutDataTypeStr=Inherit: Inherit via back propagation
  Integrator : ctrl_lib/Integrator  ts=ts  max_lim=1e6  min_lim=-1e6
  Integrator1 : ctrl_lib/Integrator  ts=ts  max_lim=1e6  min_lim=-1e6
  Product : Product  OutDataTypeStr=Inherit: Same as first input
  Sign : Signum
  Sqrt : Sqrt  SaturateOnIntegerOverflow=on
  DiffOut : Outport
  wires:
  Add/1 -> Abs/1, Sign/1
  Product/1 -> Gain1/1
  Integrator/1 -> Gain2/1
  Gain1/1 -> Add1/1
  Abs/1 -> Sqrt/1
  DiffIn/1 -> Add/1
  Add1/1 -> DiffOut/1, Integrator1/1
  Sqrt/1 -> Product/1
  Sign/1 -> Product/2, Integrator/1
  Integrator1/1 -> Add/2
  Gain2/1 -> Add1/2

== system ctrl/ctrl_slow/MtrCtrl/scale_tgt/encoder_quant ==
  tgt_in : Inport
  Constant : Constant  Value=EncResDeg
  Product : Product  Inputs=*/
  Product1 : Product  Inputs=**
  Round : Rounding  Operator=round
  tgt_out : Outport
  wires:
  tgt_in/1 -> Product/1
  Constant/1 -> Product1/2, Product/2
  Product/1 -> Round/1
  Round/1 -> Product1/1
  Product1/1 -> tgt_out/1

== stateflow chart ctrl/ctrl_fast/AutoCalMgr/autotune ==
  state init_outputs
    entry, during:
    status = AutoCalSt.NotStarted;
    vout = 0;
    Lest = -1;
    Rest = -1;
    KTrqEst = -1;
    ifbk_ofs = 0;
  state autocal_in_progress
    state ifbk_offset_id
      state ifbk_offset_cal
        entry:
        status = AutoCalSt.IfbkOfsID;
        cycle_cnt = 0;
        vout = 0;
        ifbk_pos = 0;
        ifbk_ofs = 0;
        during:
        ifbk_pos += ifbk;
        cycle_cnt++;
      state ifbk_offset_calc
        entry:
        ifbk_ofs = ifbk_pos / Cfg_OfsIDCntThshld;
      ifbk_offset_cal -> ifbk_offset_calc : [cycle_cnt >= Cfg_OfsIDCntThshld]
    state inductance_id
      state inductance_switching
        entry:
        status = AutoCalSt.IndID;
        ind_id_cnt = 0;
        cycle_cnt = 0;
        ifbk_pos = 0;
        ifbk_neg = 0;
        during:
        cycle_cnt++;
        state off_cycle
          entry:
          vout = -Cfg_IndIDMtrVin;
          ifbk_pos += ifbk;
        state on_cycle
          entry:
          vout = Cfg_IndIDMtrVin;
          ifbk_neg += ifbk;
          ind_id_cnt++;
        (default) -> on_cycle
        on_cycle -> off_cycle : [after(Cfg_IndIDSwTicks, tick)]
        off_cycle -> on_cycle : [after(Cfg_IndIDSwTicks, tick)]
      state inductance_calc
        entry:
        Lest =  Cfg_IndIDMtrVin * Cfg_IndIDTs / ((ifbk_pos - ifbk_neg) / ind_id_cnt);
        vout = 0;
        status = AutoCalSt.IndIDCoolDown;
      inductance_switching -> inductance_calc : [cycle_cnt >= Cfg_IndIDCntThshld]
    state resistance_id
      state resistance_id_on
        entry:
        status = AutoCalSt.ResID;
        ifbk_pos = 0;
        cycle_cnt = 0;
        vout = Cfg_ResIDMtrVin;
        during:
        ifbk_max = max(ifbk_max, ifbk);
        cycle_cnt++;
      state resistance_calc
        entry:
        Rest = Cfg_ResIDMtrVin / ifbk_max;
        vout = Cfg_TrqCnstIDMtrVin;
      resistance_id_on -> resistance_calc : [cycle_cnt >= Cfg_ResIDCntThshld]
    state motor_inertia_id
      entry:
      status = AutoCalSt.InertiaID;
      state motor_accel_wait
        entry:
        vout = Cfg_TrqCnstIDMtrVin;
        status = AutoCalSt.IndIDCoolDown;
        cycle_cnt = 1;
        JEst = 0;
        during:
        JEst += (- KFrcEst * spd + KTrqEst * ifbk) * TsFast;
      state motor_inertia_calc
        entry:
        vout = 0;
        JEst = JEst / spd;
      motor_accel_wait -> motor_inertia_calc : [spd >= 0.6321 * SpdMax]
    state motor_constant_id
      entry:
      status = AutoCalSt.TrqCnstID;
      cycle_cnt = 0;
      spd_max = 0;
      ifbk_pos = 0;
      state max_spd_calc
        during:
        spd_max += spd;
        ifbk_pos += ifbk;
        cycle_cnt++;
      state trq_cnst_calc
        entry:
        spd_max = spd_max / Cfg_TrqCnstIDCntThshld;
        ifbk_pos = ifbk_pos / Cfg_TrqCnstIDCntThshld;
        KTrqEst = (Cfg_TrqCnstIDMtrVin - Rest * ifbk_pos) / spd_max;
        KFrcEst = KTrqEst * ifbk_pos / spd_max;
        SpdMax = spd_max;
        IfbkMax = ifbk_max;
        IfbkSteady = ifbk_pos;
        vout = 0;
      max_spd_calc -> trq_cnst_calc : [cycle_cnt > Cfg_TrqCnstIDCntThshld]
    trq_cnst_calc -> inductance_switching : [after(Cfg_ResIDCoolDownTicks, tick) && (spd < 10.)]
    ifbk_offset_calc -> resistance_id_on
    inductance_calc -> motor_accel_wait : [after(Cfg_IndIDCoolDownTicks, tick) && spd < 5.]
    resistance_calc -> max_spd_calc : [after(Cfg_ResIDCoolDownTicks, tick)]
  state time_cnst_id [commented out]
    entry:
    status = AutoCalSt.IndID;
    cycle_cnt = 0;
    Lest = 0;
    ind_id_cnt = 0;
    state ind_id_sw_on [commented out]
      entry:
      vout = Cfg_IndIDMtrVin;
      Lest += cycle_cnt * TsFast * Rest;
      cycle_cnt = 0;
      ind_id_cnt++;
      during:
      cycle_cnt++;
    state time_cnst_wait_for_ifbk [commented out]
      entry:
      vout = -Cfg_IndIDMtrVin
      Lest += cycle_cnt * TsFast * Rest;
      cycle_cnt = 0;
      ind_id_cnt++;
      during:
      cycle_cnt++;
    time_cnst_wait_for_ifbk -> ind_id_sw_on [commented out] : [ifbk <= -ifbk_max * 0.632f]
    ind_id_sw_on -> time_cnst_wait_for_ifbk [commented out] : [ifbk >= ifbk_max * 0.632f]
  state autocal_done
    entry:
    status = AutoCalSt.Done;
    vout = 0;
  (default) -> init_outputs
  init_outputs -> ifbk_offset_cal : [Cfg_AutoCalEnbl]
  motor_inertia_calc -> autocal_done
  data: spd input single size=1; status output Enum: AutoCalSt size=1 =AutoCalSt.NotStarted; cycle_cnt local int32 size=1 =0; ifbk input single size=1; vout output single size=1 =0; ifbk_neg local single size=1 =0; ifbk_pos local single size=1 =0; Cfg_IndIDCntThshld parameter; Lest output single size=1 =-1; Cfg_ResIDCntThshld parameter; Rest output single size=1 =-1; Cfg_IndIDMtrVin parameter; Cfg_IndIDCoolDownTicks parameter; Cfg_IndIDSwTicks parameter; Cfg_IndIDTs parameter; Cfg_ResIDMtrVin parameter; Cfg_IndIDMaxThshld parameter; Cfg_IndIDMinThshld parameter; Cfg_ResIDMinThshld parameter; Cfg_ResIDMaxThshld parameter; Cfg_OfsIDCntThshld parameter; Cfg_AutoCalEnbl parameter; TsFast parameter; Cfg_ResIDCoolDownTicks parameter; spd_max local single size=1 =0; KTrqEst output single size=1 =-1; ifbk_ofs output single size=1 =-1; Cfg_TrqCnstIDCntThshld parameter; Cfg_TrqCnstIDMtrVin parameter; ifbk_max local single size=1 =0; ind_id_cnt local int32 size=1 =0; KFrcEst output single size=1 =-1; JEst output single size=1 =-1; IfbkSteady output single size=1 =-1; IfbkMax output single size=1 =-1; SpdMax output single size=1 =-1
